simulink model "ModelADabThesisBg2"  (Simulink 6.3)
settings: Solver=ode45  StartTime=0.0  StopTime=0.35  RelTol=1e-3
values from neighbouring files (symbols this model uses):
  a1 = rs*lr/(ls*lr-M^2)    (= 89.616693567)    [DateModelAD.m]
  a2 = rs*M/(ls*lr-M^2)    (= 81.4445986029)    [DateModelAD.m]
  a3 = rr*M/(ls*lr-M^2)    (= 86.6917296054)    [DateModelAD.m]
  a4 = rr*ls/(ls*lr-M^2)    (= 91.9339948833)    [DateModelAD.m]
  a5 = p/jr    (= 202.702702703)    [DateModelAD.m]
  a6 = 3*p*M/(2*(ls*lr-M^2))    (= 102.661258743)    [DateModelAD.m]
  a7 = lr/(ls*lr-M^2)    (= 25.1027152849)    [DateModelAD.m]
  a8 = M/(ls*lr-M^2)    (= 22.813613054)    [DateModelAD.m]
  p = 3    [DateModelAD.m]
libraries: powerlib_extras x1
settings Model: LastModifiedBy=LT Phyo Mg Mg  StrictBusMsg=None
settings OptimizationCC: InlineInvariantSignals=on

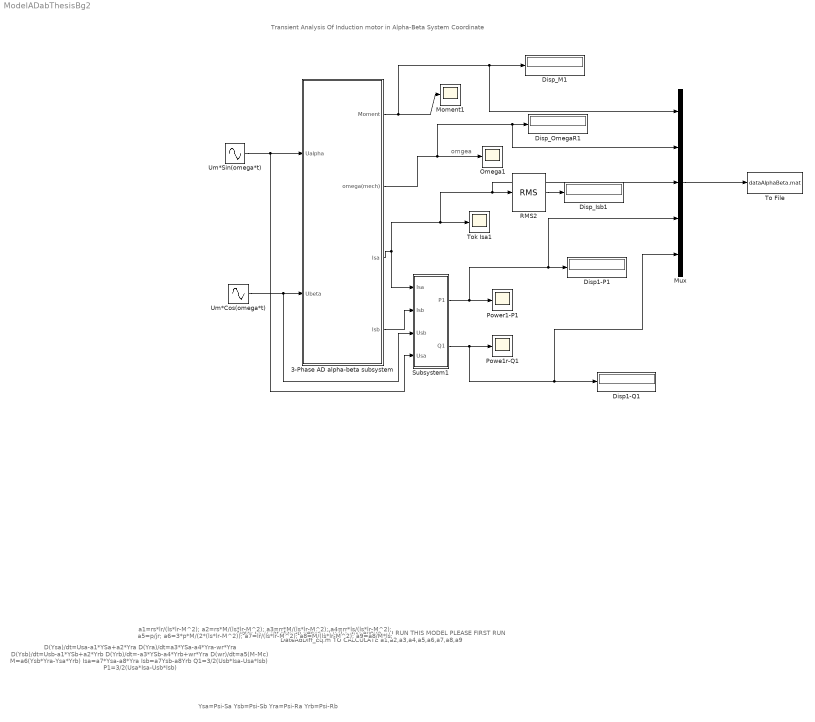
== system ModelADabThesisBg2 ==
  note: omgea
  note: Note: Only for Matlab Version 7.0.0.1 and above,
      |
      | TO RUN THIS MODEL PLEASE FIRST RUN
      | DateAdDiff_Eq.m
      | TO CALCULATE a1,a2,a3,a4,a5,a6,a7,a8,a9
  note: D(Ysa)/dt=Usa-a1*YSa+a2*Yra
      | D(Yra)/dt=a3*YSa-a4*Yra-wr*Yra
      | D(Ysb)/dt=Usb-a1*YSb+a2*Yrb
      | D(Yrb)/dt=-a3*YSb-a4*Yrb+wr*Yra
      | D(wr)/dt=a5(M-Mc)
      | M=a6(Ysb*Yra-Ysa*Yrb)
      | Isa=a7*Ysa-a8*Yra
      | Isb=a7Ysb-a8Yrb
      | Q1=3/2(Usb*Isa-Usa*Isb)
      | P1=3/2(Usa*Isa-Usb*Isb)
  note: Ysa=Psi-Sa
      | Ysb=Psi-Sb
      | Yra=Psi-Ra
      | Yrb=Psi-Rb
  note: a1=rs*lr/(ls*lr-M^2);
      | a2=rs*M/(ls*lr-M^2);
      | a3=rr*M/(ls*lr-M^2);
      | a4=rr*ls/(ls*lr-M^2);
      | a5=p/jr;
      | a6=3*p*M/(2*(ls*lr-M^2));
      | a7=lr/(ls*lr-M^2);
      | a8=M/(ls*lr-M^2);
      | a9=a8/M*ls;
  note: Transient Analysis Of Induction motor in Alpha-Beta System Coordinate
  3-Phase AD alpha-beta subsystem : Subsystem
  Disp1-P1 : Display
  Disp1-Q1 : Display
  Disp_Isb1 : Display
  Disp_M1 : Display
  Disp_OmegaR1 : Display
  Moment1 : Scope
      settings: SaveName=ScopeData9
  Mux : Mux  Inputs=5
  Omega1 : Scope
      settings: SaveName=ScopeData10
  Powe1r-Q1 : Scope
      settings: SaveName=ScopeData13
  Power1-P1 : Scope
      settings: SaveName=ScopeData12
  RMS2 : powerlib_extras/Measurements/RMS  f1=60
  Subsystem1 : Subsystem
  To File : ToFile  Filename=dataAlphaBeta.mat
  Tok Isa1 : Scope
      settings: SaveName=ScopeData11
  "Um*Cos(omega*t) " : Sin  Amplitude=311.12  Frequency=314  Phase=pi/2  SampleTime=0
  Um*Sin(omega*t) : Sin  Amplitude=-311.12  Frequency=314  SampleTime=0
  wires:
  3-Phase AD alpha-beta subsystem/3(Isa) -> Subsystem1/1(Isa), Tok Isa1/1, RMS2/1, Mux/3
  Um*Sin(omega*t)/1 -> 3-Phase AD alpha-beta subsystem/1(Ualpha), Subsystem1/4(Usa)
  "Um*Cos(omega*t) "/1 -> 3-Phase AD alpha-beta subsystem/2(Ubeta), Subsystem1/3(Usb)
  Subsystem1/1(P1) -> Power1-P1/1, Disp1-P1/1, Mux/4
  Subsystem1/2(Q1) -> Powe1r-Q1/1, Disp1-Q1/1, Mux/5
  RMS2/1 -> Disp_Isb1/1
  3-Phase AD alpha-beta subsystem/1(Moment) -> Moment1/1, Disp_M1/1, Mux/1
  3-Phase AD alpha-beta subsystem/4(Isb) -> Subsystem1/2(Isb)
  3-Phase AD alpha-beta subsystem/2(omega(mech)) -> Omega1/1, Disp_OmegaR1/1, Mux/2
  Mux/1 -> To File/1

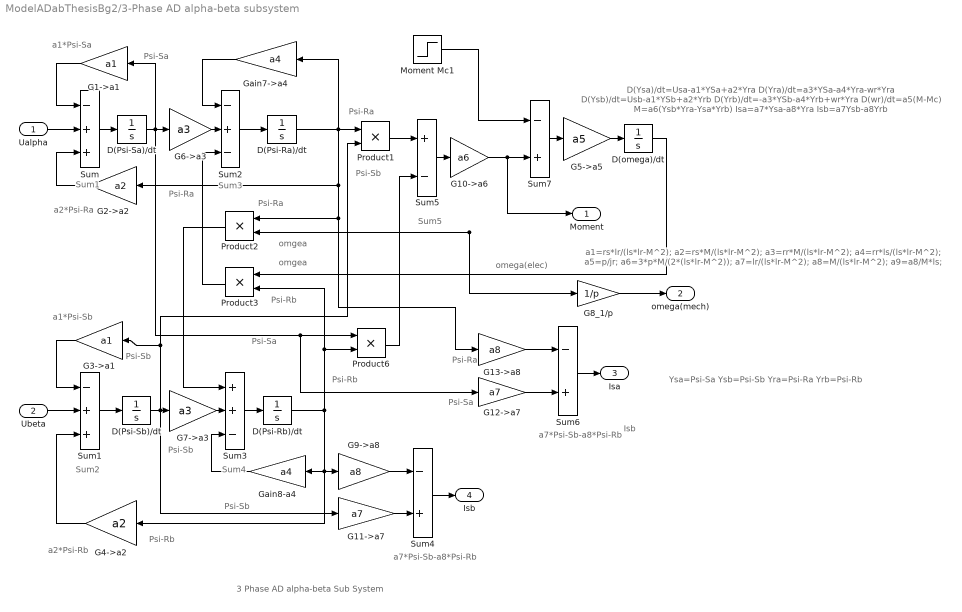
== system ModelADabThesisBg2/3-Phase AD alpha-beta subsystem ==
  note: Sum3
  note: Sum4
  note: Sum5
  note: a7*Psi-Sb-a8*Psi-Rb
  note: Sum1
  note: Sum2
  note: Psi-Sa
  note: Psi-Sa
  note: Psi-Ra
  note: Psi-Ra
  note: omgea
  note: omgea
  note: Psi-Rb
  note: Psi-Rb
  note: Psi-Rb
  note: Psi-Sb
  note: Psi-Sb
  note: Psi-Sb
  note: a1*Psi-Sa
  note: Psi-Ra
  note: a2*Psi-Ra
  note: a1*Psi-Sb
  note: a2*Psi-Rb
  note: Psi-Sb
  note: a7*Psi-Sb-a8*Psi-Rb
  note: Psi-Ra
  note: Psi-Sa
  note: Isb
  note: omega(elec)
  note: D(Ysa)/dt=Usa-a1*YSa+a2*Yra
      | D(Yra)/dt=a3*YSa-a4*Yra-wr*Yra
      | D(Ysb)/dt=Usb-a1*YSb+a2*Yrb
      | D(Yrb)/dt=-a3*YSb-a4*Yrb+wr*Yra
      | D(wr)/dt=a5(M-Mc)
      | M=a6(Ysb*Yra-Ysa*Yrb)
      | Isa=a7*Ysa-a8*Yra
      | Isb=a7Ysb-a8Yrb
  note: a1=rs*lr/(ls*lr-M^2);
      | a2=rs*M/(ls*lr-M^2);
      | a3=rr*M/(ls*lr-M^2);
      | a4=rr*ls/(ls*lr-M^2);
      | a5=p/jr;
      | a6=3*p*M/(2*(ls*lr-M^2));
      | a7=lr/(ls*lr-M^2);
      | a8=M/(ls*lr-M^2);
      | a9=a8/M*ls;
  note: Ysa=Psi-Sa
      | Ysb=Psi-Sb
      | Yra=Psi-Ra
      | Yrb=Psi-Rb
  note: 3 Phase AD alpha-beta Sub System
  Ualpha : Inport
  Ubeta : Inport  Port=2
  "D(Psi-Ra)/dt " : Integrator
  "D(Psi-Rb)/dt " : Integrator
  D(Psi-Sa)/dt : Integrator
  "D(Psi-Sb)/dt " : Integrator
  D(omega)/dt : Integrator
  G1->a1 : Gain  Orientation=left  Gain=a1
  G10->a6 : Gain  Gain=a6
  G11->a7 : Gain  Gain=a7
  G12->a7 : Gain  Gain=a7
  G13->a8 : Gain  Gain=a8
  G2->a2 : Gain  Orientation=left  Gain=a2
  G3->a1 : Gain  Orientation=left  Gain=a1
  G4->a2 : Gain  Orientation=left  Gain=a2
  G5->a5 : Gain  Gain=a5
  G6->a3 : Gain  Gain=a3
  G7->a3 : Gain  Gain=a3
  G8_1/p : Gain  Gain=1/p
  G9->a8 : Gain  Gain=a8
  Gain7->a4 : Gain  Orientation=left  Gain=a4
  Gain8-a4 : Gain  Orientation=left  Gain=a4
  Moment Mc1 : Step  Time=0.08  After=17  SampleTime=0
  Product1 : Product  RndMeth=Zero
  Product2 : Product  Orientation=left  RndMeth=Zero
  Product3 : Product  Orientation=left  RndMeth=Zero
  Product6 : Product  RndMeth=Zero
  Sum : Sum  Inputs=-++
  Sum1 : Sum  Inputs=-++
  Sum2 : Sum  Inputs=-+-
  Sum3 : Sum  Inputs=++-
  Sum4 : Sum  Inputs=-+
  Sum5 : Sum  Inputs=+-
  Sum6 : Sum  Inputs=-+
  Sum7 : Sum  Inputs=-+
  Moment : Outport
  omega(mech) : Outport  Port=2
  Isa : Outport  Port=3
  Isb : Outport  Port=4
  wires:
  Moment Mc1/1 -> Sum7/1
  Sum/1 -> D(Psi-Sa)/dt/1
  G1->a1/1 -> Sum/1
  G2->a2/1 -> Sum/3
  G3->a1/1 -> Sum1/1
  G4->a2/1 -> Sum1/3
  D(Psi-Sa)/dt/1 -> G6->a3/1, Product6/1, G12->a7/1, G1->a1/1
  "D(Psi-Sb)/dt "/1 -> G7->a3/1, G3->a1/1, Product1/2, G11->a7/1
  Sum1/1 -> "D(Psi-Sb)/dt "/1
  G7->a3/1 -> Sum3/2
  G6->a3/1 -> Sum2/2
  Sum3/1 -> "D(Psi-Rb)/dt "/1
  Gain7->a4/1 -> Sum2/1
  Sum2/1 -> "D(Psi-Ra)/dt "/1
  "D(Psi-Ra)/dt "/1 -> Product1/1, G2->a2/1, Product2/1, G13->a8/1, Gain7->a4/1
  Product3/1 -> Sum2/3
  "D(Psi-Rb)/dt "/1 -> Gain8-a4/1, G4->a2/1, G9->a8/1, Product6/2, Product3/2
  Gain8-a4/1 -> Sum3/3
  G9->a8/1 -> Sum4/1
  G11->a7/1 -> Sum4/2
  Product1/1 -> Sum5/1
  Product6/1 -> Sum5/2
  Sum5/1 -> G10->a6/1
  G10->a6/1 -> Sum7/2, Moment/1
  Sum7/1 -> G5->a5/1
  G5->a5/1 -> D(omega)/dt/1
  D(omega)/dt/1 -> Product2/2, Product3/1, G8_1/p/1
  Product2/1 -> Sum3/1
  G13->a8/1 -> Sum6/1
  G12->a7/1 -> Sum6/2
  Ualpha/1 -> Sum/2
  Ubeta/1 -> Sum1/2
  Sum6/1 -> Isa/1
  Sum4/1 -> Isb/1
  G8_1/p/1 -> omega(mech)/1

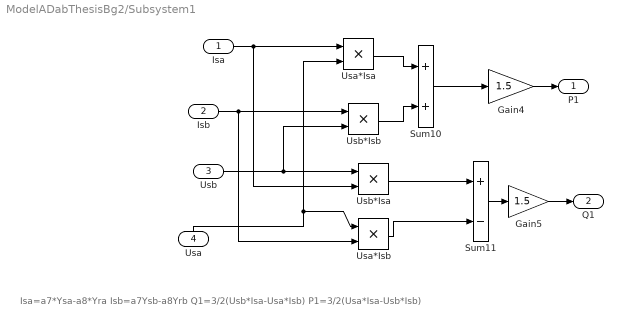
== system ModelADabThesisBg2/Subsystem1 ==
  note: Isa=a7*Ysa-a8*Yra
      | Isb=a7Ysb-a8Yrb
      | Q1=3/2(Usb*Isa-Usa*Isb)
      | P1=3/2(Usa*Isa-Usb*Isb)
  Isa : Inport
  Isb : Inport  Port=2
  Usb : Inport  Port=3
  Usa : Inport  Orientation=up  Port=4
  Gain4 : Gain  Gain=1.5
  Gain5 : Gain  Gain=1.5
  Sum10 : Sum
  Sum11 : Sum  Inputs=+-
  Usa*Isa : Product  RndMeth=Zero
  Usa*Isb : Product  RndMeth=Zero
  Usb*Isa : Product  RndMeth=Zero
  Usb*Isb : Product  RndMeth=Zero
  P1 : Outport
  Q1 : Outport  Port=2
  wires:
  Isb/1 -> Usa*Isb/2, Usb*Isb/1
  Usa*Isa/1 -> Sum10/1
  Usb*Isb/1 -> Sum10/2
  Sum10/1 -> Gain4/1
  Sum11/1 -> Gain5/1
  Usb*Isa/1 -> Sum11/1
  Usa*Isb/1 -> Sum11/2
  Usb/1 -> Usb*Isb/2, Usb*Isa/1
  Usa/1 -> Usa*Isa/2, Usa*Isb/1
  Isa/1 -> Usa*Isa/1, Usb*Isa/2
  Gain4/1 -> P1/1
  Gain5/1 -> Q1/1
